simulink model "simulate_robot_and_controller2DOF_torque"  (Simulink 9.1)
settings: Solver=ode45  StartTime=0.0  StopTime=1.0  FixedStep=0.005  RelTol=1e-3  EnableMultiTasking=on
undefined symbols (not defined in the file or in its folder): call_direct_dynamics_2dofplanar_s5b, call_inverse_dynamics_2dofplanar_s5b, call_third_order_planner
settings Model: SuppressorTable=22 serialization::archive 11 0 6 0 0 0 0 0  Creator=arturo  LastModifiedBy=arturogilaparicio
settings DataIOCC: SignalLoggingSaveFormat=ModelDataLogs
settings OptimizationCC: ExpressionDepthLimit=2147483647
settings DebuggingCC: SolverPrmCheckMsg=warning  FcnCallInpInsideContextMsg=warning  StateNameClashWarn=warning
settings SFSimCC: SimParseCustomCode=off
settings GRTTargetCC: GeneratePreprocessorConditionals=Disable all

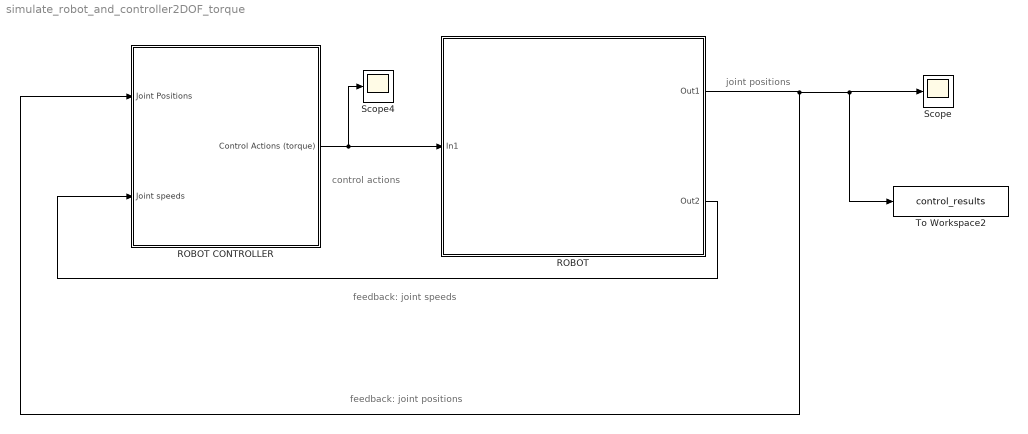
== system simulate_robot_and_controller2DOF_torque ==
  note: control actions
  note: feedback: joint positions
  note: joint positions
  note: feedback: joint speeds
  ROBOT : Subsystem
      mask Display: image(imread('images/robot2dof.png'))
  ROBOT CONTROLLER : Subsystem  Description=ROBOT CONTROLLER
      mask Display: image(imread('images/robot-controller.jpg'))
  Scope : Scope
  Scope4 : Scope
  To Workspace2 : ToWorkspace  VariableName=control_results  SampleTime=-1
  wires:
  ROBOT CONTROLLER/1(Control Actions (torque)) -> ROBOT/1(In1), Scope4/1
  ROBOT/1(Out1) -> To Workspace2/1, Scope/1, ROBOT CONTROLLER/1(Joint Positions)
  ROBOT/2(Out2) -> ROBOT CONTROLLER/2(Joint speeds)

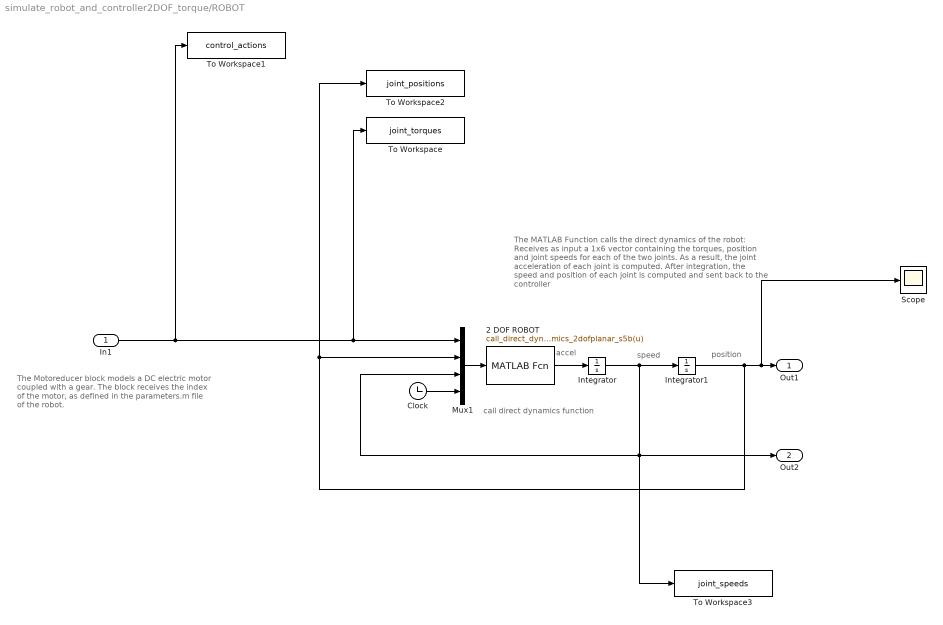
== system simulate_robot_and_controller2DOF_torque/ROBOT ==
  note: accel
  note: speed
  note: position
  note: The MATLAB Function calls the direct dynamics of the robot:
      | Receives as input a 1x6 vector containing the
      | torques, position and joint
      | speeds for each of the two joints. As a result, the joint
      | acceleration of each joint is computed.
      | After integration, the speed and position of each joint
      | is computed and sent back to the controller
  note: call direct dynamics
      |  function
  note: The Motoreducer block models a DC
      | electric motor coupled with a gear.
      | The block receives the index of the motor,
      | as defined in the parameters.m file of the robot.
  In1 : Inport
  2 DOF ROBOT : MATLABFcn  MATLABFcn=call_direct_dynamics_2dofplanar_s5b(u)  OutputDimensions=2
  Clock : Clock
  Integrator : Integrator  InitialCondition=[0 0 ]
  Integrator1 : Integrator  InitialCondition=[0 0]
  Mux1 : Mux
  Scope : Scope
  To Workspace : ToWorkspace  VariableName=joint_torques  SampleTime=-1
  To Workspace1 : ToWorkspace  VariableName=control_actions  SampleTime=-1
  To Workspace2 : ToWorkspace  VariableName=joint_positions  SampleTime=-1
  To Workspace3 : ToWorkspace  VariableName=joint_speeds  SampleTime=-1
  Out1 : Outport
  Out2 : Outport  Port=2
  wires:
  Mux1/1 -> 2 DOF ROBOT/1
  2 DOF ROBOT/1 -> Integrator/1
  Integrator/1 -> Integrator1/1, Out2/1, To Workspace3/1, Mux1/3
  Integrator1/1 -> Scope/1, Out1/1, Mux1/2, To Workspace2/1
  In1/1 -> Mux1/1, To Workspace/1, To Workspace1/1
  Clock/1 -> Mux1/4

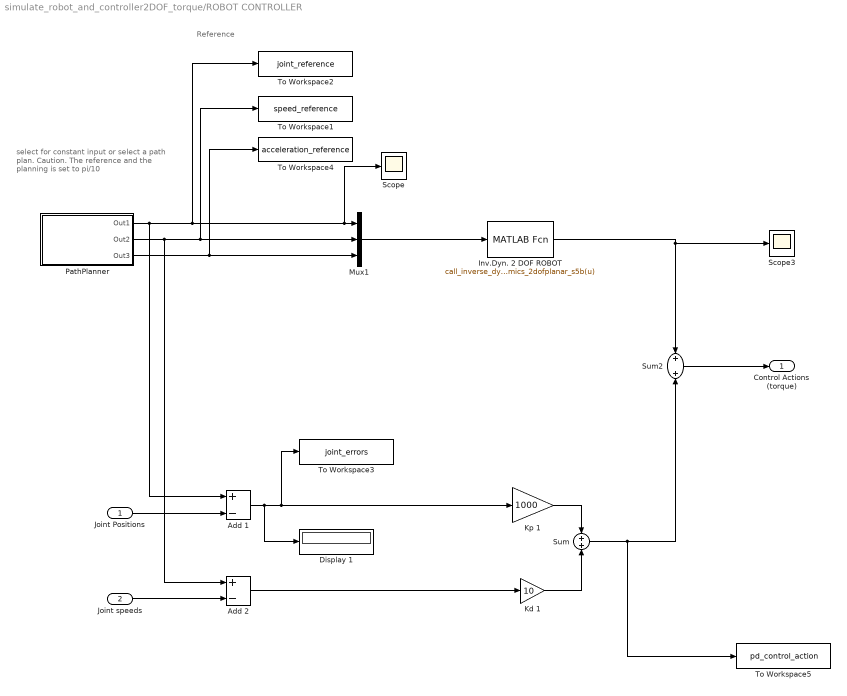
== system simulate_robot_and_controller2DOF_torque/ROBOT CONTROLLER ==
  note: Reference
  note: select for constant input or select
      | a path plan. Caution. The reference and
      | the planning is set to pi/10
  Joint Positions : Inport
  Joint speeds : Inport  Port=2
  Add 1 : Sum  Inputs=+-
  Add 2 : Sum  Inputs=+-
  Display 1 : Display
  Inv.Dyn. 2 DOF ROBOT : MATLABFcn  MATLABFcn=call_inverse_dynamics_2dofplanar_s5b(u)  OutputDimensions=2
  Kd 1 : Gain  Gain=10
  Kp 1 : Gain  Gain=1000
  Mux1 : Mux  Inputs=3
  PathPlanner : Subsystem
      mask Display: port_label('output', 1, 'q, qd, qdd')
  Scope : Scope
  Scope3 : Scope
  Sum : Sum
  Sum2 : Sum
  To Workspace1 : ToWorkspace  VariableName=speed_reference  SampleTime=-1
  To Workspace2 : ToWorkspace  VariableName=joint_reference  SampleTime=-1
  To Workspace3 : ToWorkspace  VariableName=joint_errors  SampleTime=-1
  To Workspace4 : ToWorkspace  VariableName=acceleration_reference  SampleTime=-1
  To Workspace5 : ToWorkspace  VariableName=pd_control_action  SampleTime=-1
  Control Actions (torque) : Outport
  wires:
  Sum2/1 -> Control Actions (torque)/1
  Joint Positions/1 -> Add 1/2
  Sum/1 -> To Workspace5/1, Sum2/2
  Kp 1/1 -> Sum/1
  Kd 1/1 -> Sum/2
  Add 1/1 -> Display 1/1, To Workspace3/1, Kp 1/1
  Mux1/1 -> Inv.Dyn. 2 DOF ROBOT/1
  PathPlanner/2(Out2) -> Add 2/1, To Workspace1/1, Mux1/2
  PathPlanner/3(Out3) -> To Workspace4/1, Mux1/3
  Inv.Dyn. 2 DOF ROBOT/1 -> Scope3/1, Sum2/1
  PathPlanner/1(Out1) -> Add 1/1, Scope/1, Mux1/1, To Workspace2/1
  Add 2/1 -> Kd 1/1
  Joint speeds/1 -> Add 2/2

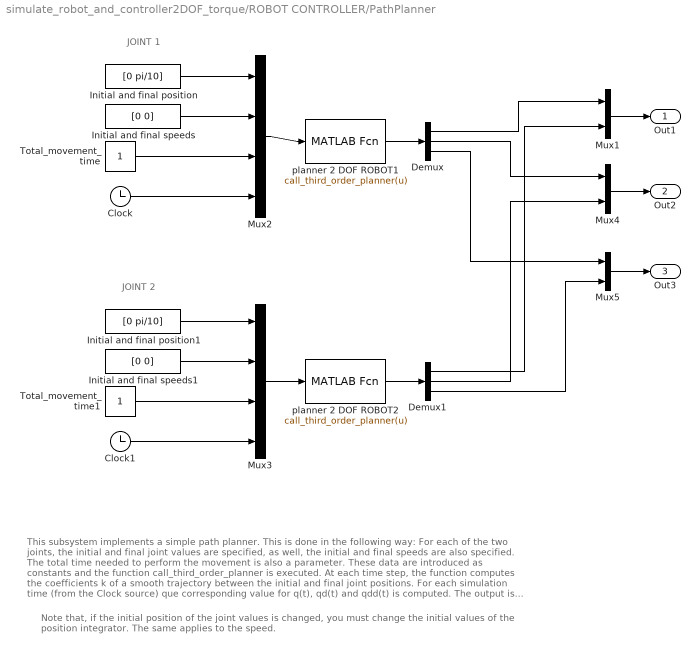
== system simulate_robot_and_controller2DOF_torque/ROBOT CONTROLLER/PathPlanner ==
  note: JOINT 1
  note: JOINT 2
  note: This subsystem implements a simple path planner. This is done in the following way: For each of the two joints,
      | the initial and final joint values are specified, as well, the initial and final speeds are also specified. The total time needed to perform the movement is also
      | a parameter. These data are introduced as constants and the function call_third_order_planner is executed. At each time step, the function computes the coefficients
      | k of a smooth trajectory between the initial and final joint positions. For each simulation time (from the Clock source) que corresponding value for q(t), qd(t) and qdd(t) is computed.
      | The output is formed by 6 variables (2 values of position, 2 of joint speed and 2 of acceleration)
  note: Note that, if the initial position of the joint values is changed, you must change the initial values of the position integrator. The same applies to the speed.
  Clock : Clock
  Clock1 : Clock
  Demux : Demux  Outputs=3
  Demux1 : Demux  Outputs=3
  Initial and final position : Constant  Value=[0 pi/10]
  Initial and final position1 : Constant  Value=[0 pi/10]
  Initial and final speeds : Constant  Value=[0 0]
  Initial and final speeds1 : Constant  Value=[0 0]
  Mux1 : Mux  Inputs=2
  Mux2 : Mux
  Mux3 : Mux
  Mux4 : Mux  Inputs=2
  Mux5 : Mux  Inputs=2
  Total_movement_time : Constant
  Total_movement_time1 : Constant
  planner 2 DOF ROBOT1 : MATLABFcn  MATLABFcn=call_third_order_planner(u)  OutputDimensions=3
  planner 2 DOF ROBOT2 : MATLABFcn  MATLABFcn=call_third_order_planner(u)  OutputDimensions=3
  Out1 : Outport
  Out2 : Outport  Port=2
  Out3 : Outport  Port=3
  wires:
  Initial and final position/1 -> Mux2/1
  Initial and final speeds/1 -> Mux2/2
  Total_movement_time/1 -> Mux2/3
  Clock/1 -> Mux2/4
  Mux2/1 -> planner 2 DOF ROBOT1/1
  Initial and final position1/1 -> Mux3/1
  Initial and final speeds1/1 -> Mux3/2
  Total_movement_time1/1 -> Mux3/3
  Clock1/1 -> Mux3/4
  Mux3/1 -> planner 2 DOF ROBOT2/1
  planner 2 DOF ROBOT1/1 -> Demux/1
  planner 2 DOF ROBOT2/1 -> Demux1/1
  Demux/1 -> Mux1/1
  Demux1/1 -> Mux1/2
  Demux/2 -> Mux4/1
  Demux1/2 -> Mux4/2
  Demux/3 -> Mux5/1
  Demux1/3 -> Mux5/2
  Mux1/1 -> Out1/1
  Mux4/1 -> Out2/1
  Mux5/1 -> Out3/1
